simulink library "pipeline_lib"  (R2015a)
settings: Solver=ode45  StartTime=0.0  StopTime=10.0  RelTol=1e-3
undefined symbols (not defined in the file or in its folder): d, L, N
undefined symbols (not defined in the file): e, P0, Q0
libraries: pipeline_lib x65, fl_lib x4, usask_hyd_ssc_lib x2
settings Model: Creator=tkw954  LastModifiedBy=tkw954
settings DebuggingCC: UnderspecifiedInitializationDetection=Classic  MergeDetectMultiDrivingBlocksExec=none  SolverPrmCheckMsg=warning  StateNameClashWarn=warning

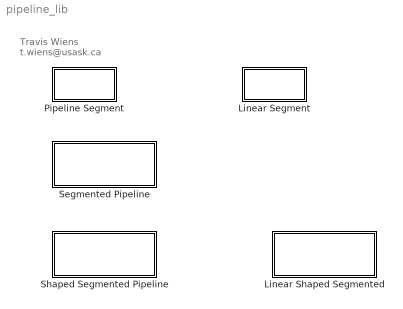
== system pipeline_lib ==
  note: Travis Wiens
      | t.wiens@usask.ca
  Linear Segment : Subsystem  mask(Segment){L=L/N, d=d, P0=P0, Q0=Q0}
      mask prompts: L "Length (m)"; d "Diameter (m)"; P0 "Initial Pressure (Pa)"; Q0 "Initial Flow (m^3/s)"
      mask help: Uses laminar flow resistance and simplified volume
  Linear Shaped Segmented : Subsystem  mask(Shaped Segmented Pipeline){N=30, x_LU=[0 1.6 2 2.5 3], d_LU=1e-3*[10 10 20 10 10], P0=0, Q0=0}
      mask prompts: N "Number of Segments"; x_LU "Shape Lookup Lengths (m)"; d_LU "Shape Lookup Diameters (m)"; P0 "Initial Pressure (Pa)"; Q0 "Initial Flow (m^3/s)"
      mask help: Implements a segmented pipeline with varying cross section, defined by lookup table.
      mask init:
      | %dimensions for autogenerated blocks
      | dx = 60;%block spacing
      | y = 30;%block verical position
      | w = 30;%block width
      | h = 30;%block height
      | 
      | x_LU=x_LU-x_LU(1);%ensure first point is 0
      | L=x_LU(end);%(m) length
      | 
      | x1=linspace(0,L,N+1);%segment intersections
      | x2=(x1(1:(end-1))+x1(2:end))/2;%segment midpoints
      | d=interp1(x_LU,d_LU,x2);%(m) interpolated diameter at midpoint of each segment
      | 
      | %delete_blocks
      | sys=gcb;
      | hcb=get_param(sys,'Handle');
      | hb=get(hcb,'blocks');
      | idx_seg=find(strncmp(hb,'segment_',8));%find segments
      | assignin('base','hb',hb)
      | assignin('base','hcb',hcb)
      | assignin('base','idx_seg',idx_seg)
      | 
      | for i=1:numel(idx_seg)
      | delete_block(sprintf('%s/%s',sys, hb{idx_seg(i)}))
      | end
      | 
      | hlines=get(hcb,'lines');
      | for i=1:numel(hlines)
      | delete_line(hlines(i).Handle)
      | end
      | 
      | %draw new segments
      | for i=1:N
      |     pos = [dx*i y+h/4 dx*i+w y+h*.75];
      |     add_block('pipeline_lib/Linear Segment',sprintf('%s/segment_%d',sys, i),'Position',pos);
      |     set_param(sprintf('%s/segment_%d',sys, i),'d',sprintf('d(%d)',i));
      | end
      | 
      | %draw connecting lines
      | if N>0
      |     add_line(sys,'A/RConn1','segment_1/LConn1','autorouting','on')
      |     add_line(sys,sprintf('segment_%d/RConn1',N),'B/RConn1','autorouting','on')
      | else
      |     add_line(sys,'A/RConn1','B/RConn1','autorouting','on')
      | end
      | 
      | for i=2:N
      |     add_line(sys,sprintf('segment_%d/RConn1',i-1),sprintf('segment_%d/LConn1', i),'autorouting','on')
      | end
      mask Display:
      | plot(x2,d)
      | plot(x2,-d)
      | for i=1:N
      |     plot(x1(i)*[1 1],d(i)*[-1 1])
      |     plot(x1(i+1)*[1 1],d(i)*[-1 1])
      | end
      | 
      | port_label('RConn', 1,'B');
      | port_label('LConn', 1,'A');
  Pipeline Segment : Subsystem  mask(Segment){L=L/N, d=d, e=e, P0=P0, Q0=Q0}
      mask prompts: L "Length (m)"; d "Diameter (m)"; e "Internal roughness (m)"; P0 "Initial Pressure (Pa)"; Q0 "Initial Flow (m^3/s)"
  Segmented Pipeline : Subsystem  mask{N=5, L=1, d=10e-3, e=1e-6, P0=0, Q0=0}
      mask prompts: N "Number of Segments"; L "Length (m)"; d "Diameter (m)"; e "Internal roughness"; P0 "Initial Pressure (Pa)"; Q0 "Initial Flow (m^3/s)"
      mask init:
      | dx = 60;
      | y = 30;
      | w = 30;
      | h = 30;
      | 
      | %delete_block
      | 
      | %hb=find_system(gcb, 'BlockType', 'Segment');
      | %hb=find_system(gcb, 'Type', 'block','FollowLinks','on');
      | %hb=find_system
      | sys=gcb;
      | hcb=get_param(sys,'Handle');
      | hb=get(hcb,'blocks');
      | idx_seg=find(strncmp(hb,'segment_',8));%find segments
      | assignin('base','hb',hb)
      | assignin('base','hcb',hcb)
      | assignin('base','idx_seg',idx_seg)
      | 
      | for i=1:numel(idx_seg)
      | delete_block(sprintf('%s/%s',sys, hb{idx_seg(i)}))
      | end
      | 
      | hlines=get(hcb,'lines');
      | for i=1:numel(hlines)
      | delete_line(hlines(i).Handle)
      | end
      | 
      | %N=2;
      | 
      | for i=1:N
      | pos = [dx*i y+h/4 dx*i+w y+h*.75];
      | add_block('pipeline_lib/Pipeline Segment',sprintf('%s/segment_%d',sys, i),'Position',pos);
      | end
      | 
      | if N>0
      | add_line(sys,'A/RConn1','segment_1/LConn1','autorouting','on')
      | add_line(sys,sprintf('segment_%d/RConn1',N),'B/RConn1','autorouting','on')
      | else
      |     add_line(sys,'A/RConn1','B/RConn1','autorouting','on')
      | end
      | 
      | for i=2:N
      |     add_line(sys,sprintf('segment_%d/RConn1',i-1),sprintf('segment_%d/LConn1', i),'autorouting','on')
      | end
  Shaped Segmented Pipeline : Subsystem  mask(Shaped Segmented Pipeline){N=30, x_LU=[0 1.6 2 2.5 3], d_LU=1e-3*[10 10 20 10 10], e=1e-6, P0=0, Q0=0}
      mask prompts: N "Number of Segments"; x_LU "Shape Lookup Lengths (m)"; d_LU "Shape Lookup Diameters (m)"; e "Internal roughness"; P0 "Initial Pressure (Pa)"; Q0 "Initial Flow (m^3/s)"
      mask help: Implements a segmented pipeline with varying cross section, defined by lookup table.
      mask init:
      | %dimensions for autogenerated blocks
      | dx = 60;%block spacing
      | y = 30;%block verical position
      | w = 30;%block width
      | h = 30;%block height
      | 
      | x_LU=x_LU-x_LU(1);%ensure first point is 0
      | L=x_LU(end);%(m) length
      | 
      | x1=linspace(0,L,N+1);%segment intersections
      | x2=(x1(1:(end-1))+x1(2:end))/2;%segment midpoints
      | d=interp1(x_LU,d_LU,x2);%(m) interpolated diameter at midpoint of each segment
      | 
      | %delete_blocks
      | sys=gcb;
      | hcb=get_param(sys,'Handle');
      | hb=get(hcb,'blocks');
      | idx_seg=find(strncmp(hb,'segment_',8));%find segments
      | assignin('base','hb',hb)
      | assignin('base','hcb',hcb)
      | assignin('base','idx_seg',idx_seg)
      | 
      | for i=1:numel(idx_seg)
      | delete_block(sprintf('%s/%s',sys, hb{idx_seg(i)}))
      | end
      | 
      | hlines=get(hcb,'lines');
      | for i=1:numel(hlines)
      | delete_line(hlines(i).Handle)
      | end
      | 
      | %draw new segments
      | for i=1:N
      |     pos = [dx*i y+h/4 dx*i+w y+h*.75];
      |     add_block('pipeline_lib/Pipeline Segment',sprintf('%s/segment_%d',sys, i),'Position',pos);
      |     set_param(sprintf('%s/segment_%d',sys, i),'d',sprintf('d(%d)',i));
      | end
      | 
      | %draw connecting lines
      | if N>0
      |     add_line(sys,'A/RConn1','segment_1/LConn1','autorouting','on')
      |     add_line(sys,sprintf('segment_%d/RConn1',N),'B/RConn1','autorouting','on')
      | else
      |     add_line(sys,'A/RConn1','B/RConn1','autorouting','on')
      | end
      | 
      | for i=2:N
      |     add_line(sys,sprintf('segment_%d/RConn1',i-1),sprintf('segment_%d/LConn1', i),'autorouting','on')
      | end
      mask Display:
      | plot(x2,d)
      | plot(x2,-d)
      | for i=1:N
      |     plot(x1(i)*[1 1],d(i)*[-1 1])
      |     plot(x1(i+1)*[1 1],d(i)*[-1 1])
      | end
      | 
      | port_label('RConn', 1,'B');
      | port_label('LConn', 1,'A');

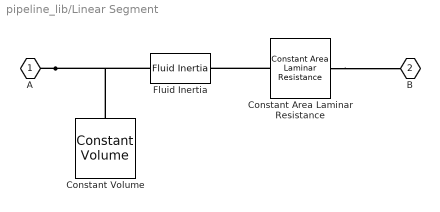
== system pipeline_lib/Linear Segment ==
  Constant Area Laminar Resistance : usask_hyd_ssc_lib/Constant Area Laminar Resistance  d=d m  L=L m  q_specify=off  q_priority=High  q=1 m^3/s  p_specify=off  p_priority=High  p=0 Pa
  Constant Volume : usask_hyd_ssc_lib/Constant Volume  V=pi/4*d^2*L m^3  p0=P0 Pa  q_specify=off  q_priority=High  q=0.001 m^3/s  p_specify=off  p_priority=High  p=0 Pa
  Fluid Inertia : fl_lib/Hydraulic/Hydraulic Elements/Fluid Inertia  area=pi/4*d^2 m^2  length=L m  q_specify=on  q_priority=High  q=Q0 m^3/s  p_specify=off  p_priority=High  p=0 Pa
  A : PMIOPort  Port=1  Side=Left
  B : PMIOPort  Port=2  Side=Right
  connections:
  Constant Area Laminar Resistance/RConn1 -- B/RConn1
  Constant Area Laminar Resistance/LConn1 -- Fluid Inertia/RConn1
  A/RConn1 -- Constant Volume/LConn1 -- Fluid Inertia/LConn1

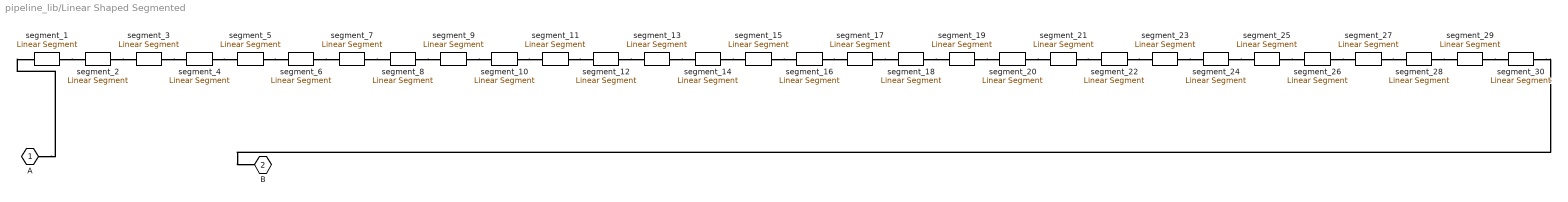
== system pipeline_lib/Linear Shaped Segmented ==
  segment_1 : pipeline_lib/Linear Segment  L=L/N  d=d(1)  P0=P0  Q0=Q0
  segment_10 : pipeline_lib/Linear Segment  L=L/N  d=d(10)  P0=P0  Q0=Q0
  segment_11 : pipeline_lib/Linear Segment  L=L/N  d=d(11)  P0=P0  Q0=Q0
  segment_12 : pipeline_lib/Linear Segment  L=L/N  d=d(12)  P0=P0  Q0=Q0
  segment_13 : pipeline_lib/Linear Segment  L=L/N  d=d(13)  P0=P0  Q0=Q0
  segment_14 : pipeline_lib/Linear Segment  L=L/N  d=d(14)  P0=P0  Q0=Q0
  segment_15 : pipeline_lib/Linear Segment  L=L/N  d=d(15)  P0=P0  Q0=Q0
  segment_16 : pipeline_lib/Linear Segment  L=L/N  d=d(16)  P0=P0  Q0=Q0
  segment_17 : pipeline_lib/Linear Segment  L=L/N  d=d(17)  P0=P0  Q0=Q0
  segment_18 : pipeline_lib/Linear Segment  L=L/N  d=d(18)  P0=P0  Q0=Q0
  segment_19 : pipeline_lib/Linear Segment  L=L/N  d=d(19)  P0=P0  Q0=Q0
  segment_2 : pipeline_lib/Linear Segment  L=L/N  d=d(2)  P0=P0  Q0=Q0
  segment_20 : pipeline_lib/Linear Segment  L=L/N  d=d(20)  P0=P0  Q0=Q0
  segment_21 : pipeline_lib/Linear Segment  L=L/N  d=d(21)  P0=P0  Q0=Q0
  segment_22 : pipeline_lib/Linear Segment  L=L/N  d=d(22)  P0=P0  Q0=Q0
  segment_23 : pipeline_lib/Linear Segment  L=L/N  d=d(23)  P0=P0  Q0=Q0
  segment_24 : pipeline_lib/Linear Segment  L=L/N  d=d(24)  P0=P0  Q0=Q0
  segment_25 : pipeline_lib/Linear Segment  L=L/N  d=d(25)  P0=P0  Q0=Q0
  segment_26 : pipeline_lib/Linear Segment  L=L/N  d=d(26)  P0=P0  Q0=Q0
  segment_27 : pipeline_lib/Linear Segment  L=L/N  d=d(27)  P0=P0  Q0=Q0
  segment_28 : pipeline_lib/Linear Segment  L=L/N  d=d(28)  P0=P0  Q0=Q0
  segment_29 : pipeline_lib/Linear Segment  L=L/N  d=d(29)  P0=P0  Q0=Q0
  segment_3 : pipeline_lib/Linear Segment  L=L/N  d=d(3)  P0=P0  Q0=Q0
  segment_30 : pipeline_lib/Linear Segment  L=L/N  d=d(30)  P0=P0  Q0=Q0
  segment_4 : pipeline_lib/Linear Segment  L=L/N  d=d(4)  P0=P0  Q0=Q0
  segment_5 : pipeline_lib/Linear Segment  L=L/N  d=d(5)  P0=P0  Q0=Q0
  segment_6 : pipeline_lib/Linear Segment  L=L/N  d=d(6)  P0=P0  Q0=Q0
  segment_7 : pipeline_lib/Linear Segment  L=L/N  d=d(7)  P0=P0  Q0=Q0
  segment_8 : pipeline_lib/Linear Segment  L=L/N  d=d(8)  P0=P0  Q0=Q0
  segment_9 : pipeline_lib/Linear Segment  L=L/N  d=d(9)  P0=P0  Q0=Q0
  A : PMIOPort  Port=1  Side=Left
  B : PMIOPort  Port=2  Side=Right
  connections:
  A/RConn1 -- segment_1/LConn1
  segment_30/RConn1 -- B/RConn1
  segment_1/RConn1 -- segment_2/LConn1
  segment_2/RConn1 -- segment_3/LConn1
  segment_3/RConn1 -- segment_4/LConn1
  segment_4/RConn1 -- segment_5/LConn1
  segment_5/RConn1 -- segment_6/LConn1
  segment_6/RConn1 -- segment_7/LConn1
  segment_7/RConn1 -- segment_8/LConn1
  segment_8/RConn1 -- segment_9/LConn1
  segment_9/RConn1 -- segment_10/LConn1
  segment_10/RConn1 -- segment_11/LConn1
  segment_11/RConn1 -- segment_12/LConn1
  segment_12/RConn1 -- segment_13/LConn1
  segment_13/RConn1 -- segment_14/LConn1
  segment_14/RConn1 -- segment_15/LConn1
  segment_15/RConn1 -- segment_16/LConn1
  segment_16/RConn1 -- segment_17/LConn1
  segment_17/RConn1 -- segment_18/LConn1
  segment_18/RConn1 -- segment_19/LConn1
  segment_19/RConn1 -- segment_20/LConn1
  segment_20/RConn1 -- segment_21/LConn1
  segment_21/RConn1 -- segment_22/LConn1
  segment_22/RConn1 -- segment_23/LConn1
  segment_23/RConn1 -- segment_24/LConn1
  segment_24/RConn1 -- segment_25/LConn1
  segment_25/RConn1 -- segment_26/LConn1
  segment_26/RConn1 -- segment_27/LConn1
  segment_27/RConn1 -- segment_28/LConn1
  segment_28/RConn1 -- segment_29/LConn1
  segment_29/RConn1 -- segment_30/LConn1

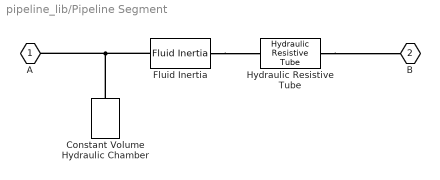
== system pipeline_lib/Pipeline Segment ==
  Constant Volume Hydraulic Chamber : fl_lib/Hydraulic/Hydraulic Elements/Constant Volume Hydraulic Chamber  ch_sp=2  wall_type=1  ch_volume=1 m^3  d_in=d m  length=L m  pr_r_coef=1.2e-12 m/Pa  time_const=0.01 s  k_sh=1.4  p_a=101325.0 Pa  flow_rate_specify=off  flow_rate_priority=High  flow_rate=0.001 m^3/s  pressure_specify=on  pressure_priority=High  pressure=P0 Pa  diameter_incr_specify=off  diameter_incr_priority=High  diameter_incr=0 m
  Fluid Inertia : fl_lib/Hydraulic/Hydraulic Elements/Fluid Inertia  area=pi/4*d^2 m^2  length=L m  q_specify=on  q_priority=High  q=Q0 m^3/s  p_specify=off  p_priority=High  p=0 Pa
  Hydraulic Resistive Tube : fl_lib/Hydraulic/Hydraulic Elements/Hydraulic Resistive Tube  cs_type=1  d_in=d m  area=1e-4 m^2  D_h=1.12e-2 m  s_factor=64  length=L m  length_ad=0 m  roughness=e m  Re_lam=2000  Re_turb=4000  length_eff=6 m  rel_roughness=0.001  q_specify=off  q_priority=High  q=0.001 m^3/s  p_specify=off  p_priority=High  p=0 Pa
  A : PMIOPort  Port=1  Side=Left
  B : PMIOPort  Port=2  Side=Right
  connections:
  Fluid Inertia/LConn1 -- Constant Volume Hydraulic Chamber/LConn1 -- A/RConn1
  Fluid Inertia/RConn1 -- Hydraulic Resistive Tube/LConn1
  Hydraulic Resistive Tube/RConn1 -- B/RConn1

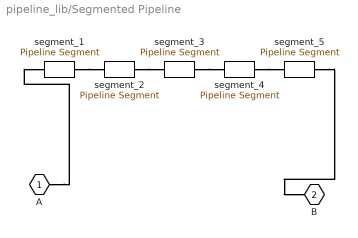
== system pipeline_lib/Segmented Pipeline ==
  segment_{1..5} (5 alike) : pipeline_lib/Pipeline Segment  L=L/N  d=d  e=e  P0=P0  Q0=Q0
  A : PMIOPort  Port=1  Side=Left
  B : PMIOPort  Port=2  Side=Right
  connections:
  A/RConn1 -- segment_1/LConn1
  segment_5/RConn1 -- B/RConn1
  segment_1/RConn1 -- segment_2/LConn1
  segment_2/RConn1 -- segment_3/LConn1
  segment_3/RConn1 -- segment_4/LConn1
  segment_4/RConn1 -- segment_5/LConn1

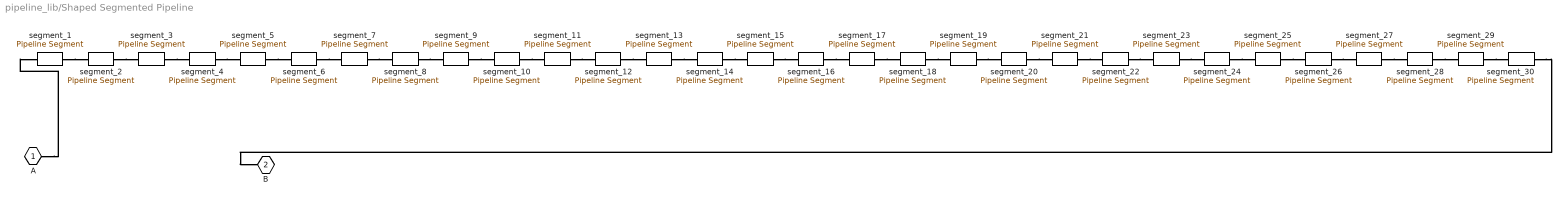
== system pipeline_lib/Shaped Segmented Pipeline ==
  segment_1 : pipeline_lib/Pipeline Segment  L=L/N  d=d(1)  e=e  P0=P0  Q0=Q0
  segment_10 : pipeline_lib/Pipeline Segment  L=L/N  d=d(10)  e=e  P0=P0  Q0=Q0
  segment_11 : pipeline_lib/Pipeline Segment  L=L/N  d=d(11)  e=e  P0=P0  Q0=Q0
  segment_12 : pipeline_lib/Pipeline Segment  L=L/N  d=d(12)  e=e  P0=P0  Q0=Q0
  segment_13 : pipeline_lib/Pipeline Segment  L=L/N  d=d(13)  e=e  P0=P0  Q0=Q0
  segment_14 : pipeline_lib/Pipeline Segment  L=L/N  d=d(14)  e=e  P0=P0  Q0=Q0
  segment_15 : pipeline_lib/Pipeline Segment  L=L/N  d=d(15)  e=e  P0=P0  Q0=Q0
  segment_16 : pipeline_lib/Pipeline Segment  L=L/N  d=d(16)  e=e  P0=P0  Q0=Q0
  segment_17 : pipeline_lib/Pipeline Segment  L=L/N  d=d(17)  e=e  P0=P0  Q0=Q0
  segment_18 : pipeline_lib/Pipeline Segment  L=L/N  d=d(18)  e=e  P0=P0  Q0=Q0
  segment_19 : pipeline_lib/Pipeline Segment  L=L/N  d=d(19)  e=e  P0=P0  Q0=Q0
  segment_2 : pipeline_lib/Pipeline Segment  L=L/N  d=d(2)  e=e  P0=P0  Q0=Q0
  segment_20 : pipeline_lib/Pipeline Segment  L=L/N  d=d(20)  e=e  P0=P0  Q0=Q0
  segment_21 : pipeline_lib/Pipeline Segment  L=L/N  d=d(21)  e=e  P0=P0  Q0=Q0
  segment_22 : pipeline_lib/Pipeline Segment  L=L/N  d=d(22)  e=e  P0=P0  Q0=Q0
  segment_23 : pipeline_lib/Pipeline Segment  L=L/N  d=d(23)  e=e  P0=P0  Q0=Q0
  segment_24 : pipeline_lib/Pipeline Segment  L=L/N  d=d(24)  e=e  P0=P0  Q0=Q0
  segment_25 : pipeline_lib/Pipeline Segment  L=L/N  d=d(25)  e=e  P0=P0  Q0=Q0
  segment_26 : pipeline_lib/Pipeline Segment  L=L/N  d=d(26)  e=e  P0=P0  Q0=Q0
  segment_27 : pipeline_lib/Pipeline Segment  L=L/N  d=d(27)  e=e  P0=P0  Q0=Q0
  segment_28 : pipeline_lib/Pipeline Segment  L=L/N  d=d(28)  e=e  P0=P0  Q0=Q0
  segment_29 : pipeline_lib/Pipeline Segment  L=L/N  d=d(29)  e=e  P0=P0  Q0=Q0
  segment_3 : pipeline_lib/Pipeline Segment  L=L/N  d=d(3)  e=e  P0=P0  Q0=Q0
  segment_30 : pipeline_lib/Pipeline Segment  L=L/N  d=d(30)  e=e  P0=P0  Q0=Q0
  segment_4 : pipeline_lib/Pipeline Segment  L=L/N  d=d(4)  e=e  P0=P0  Q0=Q0
  segment_5 : pipeline_lib/Pipeline Segment  L=L/N  d=d(5)  e=e  P0=P0  Q0=Q0
  segment_6 : pipeline_lib/Pipeline Segment  L=L/N  d=d(6)  e=e  P0=P0  Q0=Q0
  segment_7 : pipeline_lib/Pipeline Segment  L=L/N  d=d(7)  e=e  P0=P0  Q0=Q0
  segment_8 : pipeline_lib/Pipeline Segment  L=L/N  d=d(8)  e=e  P0=P0  Q0=Q0
  segment_9 : pipeline_lib/Pipeline Segment  L=L/N  d=d(9)  e=e  P0=P0  Q0=Q0
  A : PMIOPort  Port=1  Side=Left
  B : PMIOPort  Port=2  Side=Right
  connections:
  A/RConn1 -- segment_1/LConn1
  segment_30/RConn1 -- B/RConn1
  segment_1/RConn1 -- segment_2/LConn1
  segment_2/RConn1 -- segment_3/LConn1
  segment_3/RConn1 -- segment_4/LConn1
  segment_4/RConn1 -- segment_5/LConn1
  segment_5/RConn1 -- segment_6/LConn1
  segment_6/RConn1 -- segment_7/LConn1
  segment_7/RConn1 -- segment_8/LConn1
  segment_8/RConn1 -- segment_9/LConn1
  segment_9/RConn1 -- segment_10/LConn1
  segment_10/RConn1 -- segment_11/LConn1
  segment_11/RConn1 -- segment_12/LConn1
  segment_12/RConn1 -- segment_13/LConn1
  segment_13/RConn1 -- segment_14/LConn1
  segment_14/RConn1 -- segment_15/LConn1
  segment_15/RConn1 -- segment_16/LConn1
  segment_16/RConn1 -- segment_17/LConn1
  segment_17/RConn1 -- segment_18/LConn1
  segment_18/RConn1 -- segment_19/LConn1
  segment_19/RConn1 -- segment_20/LConn1
  segment_20/RConn1 -- segment_21/LConn1
  segment_21/RConn1 -- segment_22/LConn1
  segment_22/RConn1 -- segment_23/LConn1
  segment_23/RConn1 -- segment_24/LConn1
  segment_24/RConn1 -- segment_25/LConn1
  segment_25/RConn1 -- segment_26/LConn1
  segment_26/RConn1 -- segment_27/LConn1
  segment_27/RConn1 -- segment_28/LConn1
  segment_28/RConn1 -- segment_29/LConn1
  segment_29/RConn1 -- segment_30/LConn1
